simulink model "sitl"  (R2025a)
settings: Solver=FixedStepAuto  StartTime=0.0  StopTime=inf  RelTol=1e-3  EnableMultiTasking=on
PreLoadFcn:
  | SampleTime = 1e-3;
  | isUsingSimulinkMixer=true;
libraries: px4Sensorslib x2, px4Peripheralslib x1
CloseFcn:
  | clear SampleTime;
settings Model: ExtModeTrigDuration=10  Creator=The MathWorks, Inc.  LastModifiedBy=aero
settings SolverCC: AlgebraicLoopSolver=TrustRegion  PositivePriorityOrder=on  MaxZcPerStep=1.0
settings OptimizationCC: EnhancedBackFolding=on  PassReuseOutputArgsAs=Individual arguments  ZeroExternalMemoryAtStartup=off  ZeroInternalMemoryAtStartup=off  MaxStackSize=64  OptimizeBlockOrder=speed  DifferentSizesBufferReuse=on  OptimizationCustomize=off  EfficientTunableParamExpr=on
settings DebuggingCC: ParameterPrecisionLossMsg=none  ParameterTunabilityLossMsg=error  UnconnectedInputMsg=warning  UnconnectedOutputMsg=warning  UnconnectedLineMsg=warning  SubsystemReferenceDiagnosticForUnitTest=warning
settings HardwareCC: ProdBitPerPointer=32.0  ProdBitPerSizeT=32.0  ProdBitPerPtrDiffT=32.0  ProdLargestAtomicInteger=Long  ProdLargestAtomicFloat=Double  ProdWordSize=32.0  ProdLongLongMode=on  ProdHWDeviceType=ARM Compatible->ARM Cortex
settings ModelReferenceCC: EnableRefExpFcnMdlSchedulingChecks=on
settings SFSimCC: MATLABDynamicMemAlloc=off  SimTargetLang=C++  SimDLTargetLibrary=mkl-dnn
settings RTWCC: SystemTargetFile=ert.tlc  HardwareBoard=PX4 Host Target  TLCOptions="-aInlineSetEventsForThisBaseRateFcn=TLC_FALSE -aSuppressMultiTaskScheduler=TLC_FALSE  -aRateBasedStepFcn=0"  TemplateMakefile=ert_default_tmf  Toolchain=GNU Tools for PX4 Autopilots  PortableWordSizes=on  TargetLang=C++  GPUComputeCapability=3.5  DLArmComputeVersion=19.05  Description=Embedded Coder
settings CodeAppCC: ForceParamTrailComments=on  IgnoreCustomStorageClasses=off  OperatorAnnotations=on  SimulinkDataObjDesc=on  SFDataObjDesc=on  InsertBlockDesc=on
settings ERTTargetCC: ExtModeTransport=2.0  InlinedParameterPlacement=Hierarchical

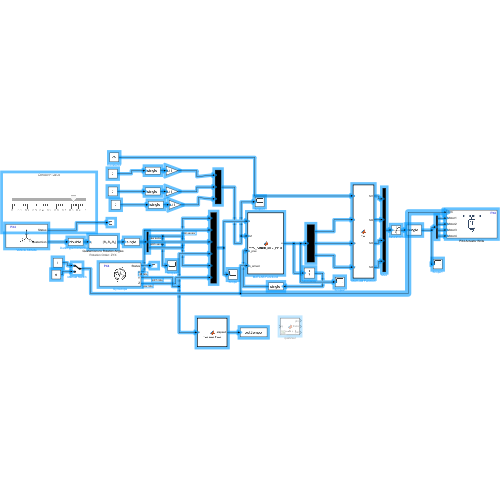
[thumbnail: Simulink's stored preview of the top-level diagram]
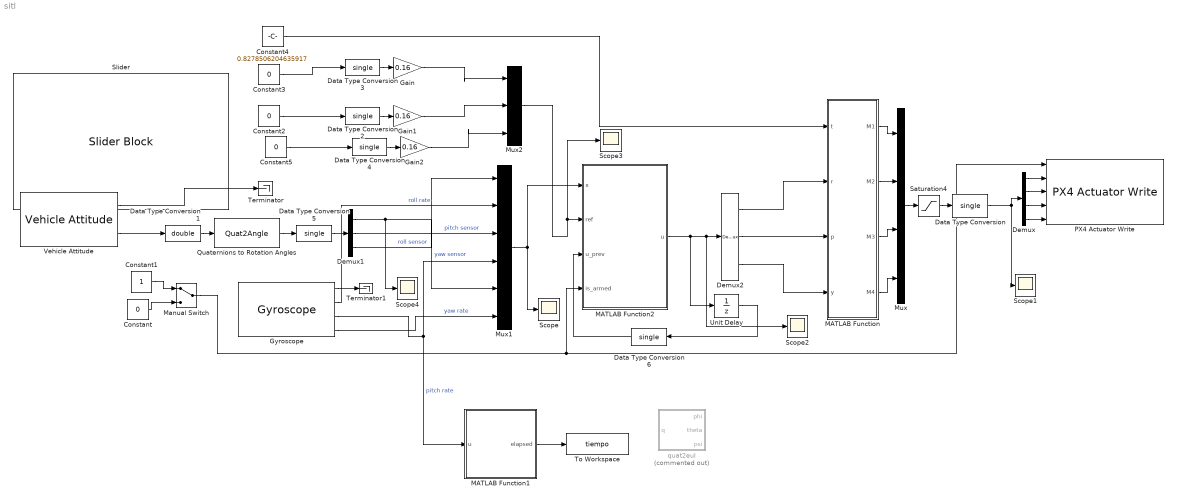
== system sitl ==
  Constant : Constant  Value=0  OutDataTypeStr=boolean
  Constant1 : Constant  OutDataTypeStr=boolean
  Constant2 : Constant  Value=0
  Constant3 : Constant  Value=0
  Constant4 : Constant  Value=0.8278506204635917
  Constant5 : Constant  Value=0
  Data Type Conversion{,2..6} (6 alike) : DataTypeConversion  OutDataTypeStr=single  SaturateOnIntegerOverflow=off  RndMeth=Floor
  Data Type Conversion1 : DataTypeConversion  OutDataTypeStr=double  SaturateOnIntegerOverflow=off  RndMeth=Floor
  Demux : Demux
  Demux1 : Demux  Outputs=3
  Demux2 : Demux  Outputs=3
  Gain : Gain  Gain=0.16
  Gain1 : Gain  Gain=0.16
  Gain2 : Gain  Gain=0.16
  Gyroscope : px4Sensorslib/Gyroscope  uorbTimeStamp=off  BlockingMode=off  BlockTimeout=1e-3  sampleTime=0.015
  MATLAB Function : MATLAB Function  TreatAsAtomicUnit=on
  MATLAB Function1 : MATLAB Function  TreatAsAtomicUnit=on
  MATLAB Function2 : MATLAB Function  TreatAsAtomicUnit=on
  Manual Switch : ManualSwitch
  Mux : Mux
  Mux1 : Mux  Inputs=6
  Mux2 : Mux  Inputs=3
  PX4 Actuator Write : px4Peripheralslib/PX4 Actuator Write  Motor1Enable=on  Motor2Enable=on  Motor3Enable=on  Motor4Enable=on  Motor5Enable=off  Motor6Enable=off  Motor7Enable=off  Motor8Enable=off  Motor9Enable=off  Motor10Enable=off  Motor11Enable=off  Motor12Enable=off  IsMotorArray=off  Servo1Enable=off  Servo2Enable=off  Servo3Enable=off  Servo4Enable=off  Servo5Enable=off  Servo6Enable=off  Servo7Enable=off  Servo8Enable=off  IsServoArray=off
  Quaternions to Rotation Angles : Quat2Angle
      settings: AttributesFormatString=Rotation Order: %<rotationOrder>
  Saturation4 : Saturate  UpperLimit=1  LowerLimit=0
  Scope{,1..4} (5 alike) : Scope
      Scope settings: ActiveDisplayYMinimum=-0.62053689360618591  ActiveDisplayYMaximum=0.55083355307579041
      Scope1 settings: ActiveDisplayYMinimum=-1.9221124811650505  ActiveDisplayYMaximum=2.19156354528468  DataLoggingVariableName=ScopeData3
      Scope2 settings: ActiveDisplayYMinimum=-0.51363188988923469  ActiveDisplayYMaximum=0.24970959563642769
      Scope3 settings: ActiveDisplayYMinimum=-1  ActiveDisplayYMaximum=1  DataLoggingVariableName=ScopeData2
      Scope4 settings: ActiveDisplayYMinimum=-0.62053689360618591  ActiveDisplayYMaximum=0.55083355307579041  DataLoggingVariableName=ScopeData4
  Slider : SliderBlock  ScaleMax=1
  Terminator : Terminator
  Terminator1 : Terminator
  To Workspace : ToWorkspace  VariableName=tiempo  SaveFormat=Timeseries  SampleTime=-1
  Unit Delay : UnitDelay  SampleTime=-1  HasFrameUpgradeWarning=on
  Vehicle Attitude : px4Sensorslib/Vehicle Attitude  rollRate=off  pitchRate=off  yawRate=off  quaternion=on  uorbTimeStamp=off  BlockingMode=off  BlockTimeout=0.001  sampleTime=0.015
  quat2eul : MATLAB Function  Commented=on  TreatAsAtomicUnit=on
  wires:
  Mux1/1 -> Scope/1, MATLAB Function2/1(x)
  Gain/1 -> Mux2/1
  Demux2/2 -> MATLAB Function/3(p)
  Gyroscope/4 -> Mux1/6  "yaw rate"
  Vehicle Attitude/1 -> Terminator/1
  Gyroscope/3 -> Mux1/4, MATLAB Function1/1(u)  "pitch rate"
  Demux2/1 -> MATLAB Function/2(r)
  Constant1/1 -> Manual Switch/1
  MATLAB Function2/1(u) -> Unit Delay/1, Scope2/1, Demux2/1
  Demux/4 -> PX4 Actuator Write/5
  Gain1/1 -> Mux2/2
  MATLAB Function/1(M1) -> Mux/1
  Mux/1 -> Saturation4/1
  Constant/1 -> Manual Switch/2
  MATLAB Function/3(M3) -> Mux/3
  MATLAB Function/4(M4) -> Mux/4
  Vehicle Attitude/2 -> Data Type Conversion1/1
  Saturation4/1 -> Data Type Conversion/1
  Demux1/1 -> Mux1/5, Scope4/1  "yaw sensor"
  Demux/1 -> PX4 Actuator Write/2
  Quaternions to Rotation Angles/1 -> Data Type Conversion5/1
  Demux/2 -> PX4 Actuator Write/3
  Constant4/1 -> MATLAB Function/1(t)
  MATLAB Function1/1(elapsed) -> To Workspace/1
  Constant3/1 -> Data Type Conversion3/1
  Data Type Conversion1/1 -> Quaternions to Rotation Angles/1
  Manual Switch/1 -> MATLAB Function2/4(is_armed), PX4 Actuator Write/1
  Data Type Conversion/1 -> Demux/1, Scope1/1
  Data Type Conversion3/1 -> Gain/1
  MATLAB Function/2(M2) -> Mux/2
  Unit Delay/1 -> Data Type Conversion6/1
  Data Type Conversion4/1 -> Gain2/1
  Gyroscope/1 -> Terminator1/1
  Gain2/1 -> Mux2/3
  Gyroscope/2 -> Mux1/2  "roll rate"
  Constant2/1 -> Data Type Conversion2/1
  Constant5/1 -> Data Type Conversion4/1
  Demux2/3 -> MATLAB Function/4(y)
  Data Type Conversion2/1 -> Gain1/1
  Demux1/3 -> Mux1/1  "roll sensor"
  Demux/3 -> PX4 Actuator Write/4
  Demux1/2 -> Mux1/3  "pitch sensor"
  Data Type Conversion5/1 -> Demux1/1
  Data Type Conversion6/1 -> MATLAB Function2/3(u_prev)
  Mux2/1 -> Scope3/1, MATLAB Function2/2(ref)

== matlab function sitl/MATLAB Function1 ==
  data: u input; elapsed output
function elapsed = measureTime(u)
% u: entrada dummy para forzar ejecución por step
%#codegen

elapsed = 0.0;   %  tipo fijo (double escalar)

coder.extrinsic('tic','toc')

persistent tStart
if isempty(tStart)
    tStart = tic;
end

elapsed = toc(tStart);
tStart = tic;

== matlab function sitl/MATLAB Function ==
  data: t input; M1 output; r input; M2 output; M3 output; M4 output; p input; y input
function [M1,M2,M3,M4]  = fcn(t,r, p, y)
M1 = t - 0.707107*r + 0.707107*p + y;
M2 = t + 0.707107*r - 0.707107*p + y;
M3 = t + 0.707107*r + 0.707107*p - y;
M4 = t - 0.707107*r - 0.707107*p - y;

== matlab function sitl/MATLAB Function2 ==
  data: x input; u output; ref input; u_prev input; is_armed input
function u = MPC_Amadi_SITL_Final(x, ref, u_prev, is_armed)
    % --- CONFIGURACIÓN DE PARÁMETROS PERSISTENTES ---
    persistent Ad Bd Cd F Phi H_inv x_old Nc Np m q n_aug M_const gamma_const
    
    % Ts debe coincidir con el Fixed-step size de tu Solver en Simulink
    Ts = single(0.02);  
    Np_val = 3; % Horizonte corto = menos oscilación lenta en SITL
    Nc_val = 2; 
    
    % --- INICIALIZACIÓN (Solo se ejecuta una vez) ---
    if isempty(Ad)
        Np = Np_val; Nc = Nc_val;
        
        % Inercias del modelo (Ajustadas para estabilidad)
        Ixx = single(0.0213); Iyy = single(0.02217); Izz = single(0.0282);
        
        % 1. Matrices Continuas
        Ac = single([0 1 0 0 0 0; 0 0 0 0 0 0; 0 0 0 1 0 0; 0 0 0 0 0 0; 0 0 0 0 0 1; 0 0 0 0 0 0]);
        Bc = single([0 0 0; 1/Ixx 0 0; 0 0 0; 0 1/Iyy 0; 0 0 0; 0 0 1/Izz]);
        Cd = single([1 0 0 0 0 0; 0 0 1 0 0 0; 0 0 0 0 1 0]);
        
        % 2. Discretización con Amortiguamiento (Damping)
        % Reducimos ligeramente los términos de velocidad (p, q, r) para frenar la oscilación
        Ad = eye(6, 'single') + Ac * Ts;
        Ad(2,2) = 0.90; % Fricción artificial en Roll rate
        Ad(4,4) = 0.90; % Fricción artificial en Pitch rate
        Ad(6,6) = 0.90; % Fricción artificial en Yaw rate
        
        Bd = Bc * Ts;
        
        % 3. Modelo Aumentado
        [n_s, n_i] = size(Bd); [n_o, ~] = size(Cd);
        m = n_i; q = n_o; n_aug = n_s + q;
        
        A_aug = [Ad, zeros(n_s, q, 'single'); Cd*Ad, eye(q, 'single')];
        B_aug = [Bd; Cd*Bd];
        C_aug = [zeros(q, n_s, 'single'), eye(q, 'single')];
        
        % 4. Matrices de Predicción F y Phi
        F = zeros(Np*q, n_aug, 'single');
        Phi = zeros(Np*q, Nc*m, 'single');
        temp_A = A_aug;
        for i = 1:Np
            F((i-1)*q+1:i*q, :) = C_aug * temp_A;
            for j = 1:Nc
                if i >= j
                    Phi((i-1)*q+1:i*q, (j-1)*m+1:j*m) = C_aug * (A_aug^(i-j)) * B_aug;
                end
            end
            temp_A = temp_A * A_aug;
        end
        
        % 5. Peso de Control (Rw) - Ajustado para SITL
        % Si el dron oscila mucho, sube este valor a 3000 o 5000
        Rw = eye(Nc*m, 'single') * 1800.0; 
        H = Phi' * Phi + Rw;
        H_inv = inv(H);
        
        % 6. Restricciones (Constraints)
        M_const = [eye(Nc*m, 'single'); -eye(Nc*m, 'single')];
        % Delta_u máximo de 0.05 para evitar saltos bruscos
        gamma_const = ones(2*Nc*m, 1, 'single') * 0.05; 
        
        x_old = zeros(6, 1, 'single'); 
    end
    
    % --- LÓGICA DE ARMADO / ANTI-WINDUP ---
    if is_armed < 0.5
        u = zeros(3, 1, 'single');
        x_old = single(x); 
        return;
    end
    
    % --- CÁLCULO EN TIEMPO REAL ---
    x_s = single(x); ref_s = single(ref); u_prev_s = single(u_prev);
    
    % Estado aumentado
    delta_x = x_s - x_old;
    x_aug = [delta_x; Cd * x_s];
    
    % Referencia sobre el horizonte
    Rs = zeros(Np*q, 1, 'single');
    for i = 1:Np; Rs((i-1)*q+1 : i*q) = ref_s; end
    
    % Optimización libre
    E_error = Rs - F * x_aug;
    f_vec = -Phi' * E_error;
    dU_free = -H_inv * f_vec;
    
    % Algoritmo de Hildreth (Si hay violación de restricciones)
    if any(M_const * dU_free > gamma_const)
        n_cons = length(gamma_const);
        lambda = zeros(n_cons, 1, 'single');
        for iter = 1:15
            lambda_prev = lambda;
            for i = 1:n_cons
                w = M_const(i,:) * H_inv * M_const(i,:)';
                la_inc = -(M_const(i,:) * dU_free - gamma_const(i)) / w;
                lambda(i) = max(0, lambda(i) + la_inc);
            end
            if norm(lambda - lambda_prev) < 1e-4; break; end
        end
        dU_opt = -H_inv * (f_vec + M_const' * lambda);
    else
        dU_opt = dU_free;
    end
    
    % Cálculo final de u y saturación de seguridad
    u_calc = u_prev_s + dU_opt(1:3);
    u = max(min(u_calc, 0.3), -0.3); % Máximo 30% de autoridad para actitud
    
    x_old = x_s;
end

== matlab function sitl/quat2eul ==
  data: q input; phi output; theta output; psi output
function [phi,theta,psi] = quat2eul(q)

% Quaternion conversion to Euler angles based on the PX4 Firmware v1.10.2
% release.

phi = atan2(2*(q(1)*q(2) + q(3)* q(4)), q(1)^2 - q(2)^2 - q(3)^2 + q(4)^2);
theta = asin(-2*(q(2)*q(4) - q(1)*q(3)));
psi = atan2(2*(q(2)*q(3) + q(1)* q(4)), q(1)^2 + q(2)^2 - q(3)^2 - q(4)^2);
end
